simulink model "VIPRStEnCtrl"  (R2018b)
settings: Solver=FixedStepDiscrete  StartTime=0.0  StopTime=10.0  FixedStep=0.01  RelTol=1e-3
undefined symbols (not defined in the file or in its folder): data, PassStFtEn_Clear, PassStFtEn_Set, SecRwRtStBkReclnEn_Clear, SecRwRtStBkReclnEn_Set, SecRwRtStFwdBkwdEn_Clear, SecRwRtStFwdBkwdEn_Set, SecRwRtStLgrstUpwdDnwdEn_Clear, SecRwRtStLgrstUpwdDnwdEn_Set, SecRwRtStLtwdRtwdEn_Clear, SecRwRtStLtwdRtwdEn_Set, ThdRwLtStBkReclnEn_Clear, ThdRwLtStBkReclnEn_Set, ThdRwLtStFwdBkwdEn_Clear, ThdRwLtStFwdBkwdEn_Set, ThdRwRtStBkReclnEn_Clear, ThdRwRtStBkReclnEn_Set, ThdRwRtStFwdBkwdEn_Clear, ThdRwRtStFwdBkwdEn_Set
libraries: simulink x1
settings Model: Creator=sn2xws  LastModifiedBy=sn2xws
settings DataIOCC: SaveFormat=StructureWithTime
settings OptimizationCC: DefaultParameterBehavior=Inlined  EnhancedBackFolding=on  PassReuseOutputArgsAs=Individual arguments  ZeroExternalMemoryAtStartup=off  ZeroInternalMemoryAtStartup=off  OptimizeBlockOrder=speed  DifferentSizesBufferReuse=on  OptimizationCustomize=off
settings DebuggingCC: ParameterTunabilityLossMsg=error
settings ModelReferenceCC: ModelReferenceNumInstancesAllowed=Single
settings SFSimCC: MATLABDynamicMemAlloc=off
settings RTWCC: SystemTargetFile=autosar.tlc  GenCodeOnly=on  TemplateMakefile=ert_default_tmf  Description=AUTOSAR  GenerateReport=on  IncludeHyperlinkInReport=on  LaunchReport=on  GenerateTraceInfo=on  GenerateTraceReport=on  GenerateTraceReportSl=on  GenerateTraceReportSf=on  GenerateTraceReportEml=on  GenerateCodeMetricsReport=on
settings CodeAppCC: ForceParamTrailComments=on  IgnoreCustomStorageClasses=off  OperatorAnnotations=on  SimulinkDataObjDesc=on  SFDataObjDesc=on  InsertBlockDesc=on
settings STFCustomTargetCC: TargetLangStandard=C99 (ISO)  MultiwordLength=256  ParMdlRefBuildCompliant=on  CompOptLevelCompliant=on  IncludeMdlTerminateFcn=off  CombineOutputUpdateFcns=on  SuppressErrorStatus=on  ERTCustomFileBanners=on  SupportNonFinite=off  SupportComplex=off  SupportContinuousTime=off  SupportNonInlinedSFcns=off  RemoveResetFunc=on  MATLABClassNameForMDSCustomization=Simulink.SoftwareTarget.ERTCustomization  AutosarCompliant=on  UseToolchainInfoCompliant=on  LookupTableObjectStructAxisOrder=2,1,3,4,...  LUTObjectStructOrderEvenSpacing=Size,Table,Breakpoints  SystemTargetFile=autosar.tlc
settings ERTTargetCC: TargetLangStandard=C99 (ISO)  ConcurrentExecutionCompliant=off  IncludeMdlTerminateFcn=off  SuppressErrorStatus=on  SupportNonFinite=off  SupportComplex=off  ModelStepFunctionPrototypeControlCompliant=off  CPPClassGenCompliant=off  AutosarCompliant=on  LookupTableObjectStructAxisOrder=2,1,3,4,...  LUTObjectStructOrderEvenSpacing=Size,Table,Breakpoints  InlinedParameterPlacement=NonHierarchical  ERTCustomFileTemplate=example_file_process.tlc  ERTFilePackagingFormat=Compact

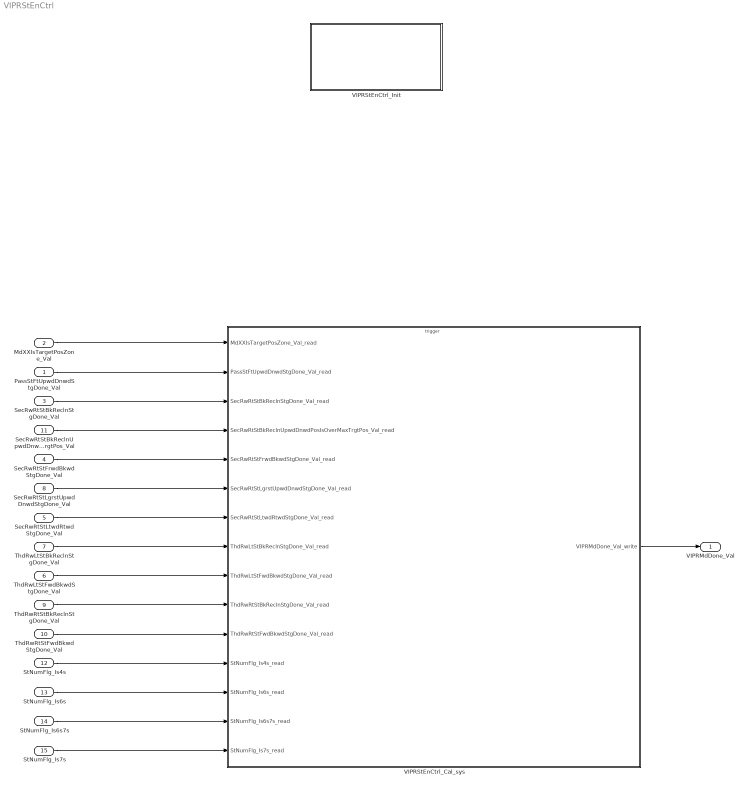
== system VIPRStEnCtrl ==
  PassStFtUpwdDnwdStgDone_Val : Inport  OutDataTypeStr=boolean  PortDimensions=1
  MdXXIsTargetPosZone_Val : Inport  Port=2  OutDataTypeStr=uint32  PortDimensions=1
  SecRwRtStBkReclnStgDone_Val : Inport  Port=3  OutDataTypeStr=boolean  PortDimensions=1
  SecRwRtStFrwdBkwdStgDone_Val : Inport  Port=4  OutDataTypeStr=boolean  PortDimensions=1
  SecRwRtStLtwdRtwdStgDone_Val : Inport  Port=5  OutDataTypeStr=boolean  PortDimensions=1
  ThdRwLtStFwdBkwdStgDone_Val : Inport  Port=6  OutDataTypeStr=boolean  PortDimensions=1
  ThdRwLtStBkReclnStgDone_Val : Inport  Port=7  OutDataTypeStr=boolean  PortDimensions=1
  SecRwRtStLgrstUpwdDnwdStgDone_Val : Inport  Port=8  OutDataTypeStr=boolean  PortDimensions=1
  ThdRwRtStBkReclnStgDone_Val : Inport  Port=9  OutDataTypeStr=boolean  PortDimensions=1
  ThdRwRtStFwdBkwdStgDone_Val : Inport  Port=10  OutDataTypeStr=boolean  PortDimensions=1
  SecRwRtStBkReclnUpwdDnwdPosIsOverMaxTrgtPos_Val : Inport  Port=11  OutDataTypeStr=boolean  PortDimensions=1
  StNumFlg_Is4s : Inport  Port=12  OutDataTypeStr=boolean  PortDimensions=1
  StNumFlg_Is6s : Inport  Port=13  OutDataTypeStr=boolean  PortDimensions=1
  StNumFlg_Is6s7s : Inport  Port=14  OutDataTypeStr=boolean  PortDimensions=1
  StNumFlg_Is7s : Inport  Port=15  OutDataTypeStr=boolean  PortDimensions=1
  VIPRStEnCtrl_Cal_sys : Subsystem
  VIPRStEnCtrl_Init : Subsystem
  VIPRMdDone_Val : Outport  OutDataTypeStr=uint8  PortDimensions=1
  wires:
  VIPRStEnCtrl_Cal_sys/1(VIPRMdDone_Val_write) -> VIPRMdDone_Val/1
  SecRwRtStBkReclnUpwdDnwdPosIsOverMaxTrgtPos_Val/1 -> VIPRStEnCtrl_Cal_sys/4(SecRwRtStBkReclnUpwdDnwdPosIsOverMaxTrgtPos_Val_read)
  MdXXIsTargetPosZone_Val/1 -> VIPRStEnCtrl_Cal_sys/1(MdXXIsTargetPosZone_Val_read)
  ThdRwRtStBkReclnStgDone_Val/1 -> VIPRStEnCtrl_Cal_sys/10(ThdRwRtStBkReclnStgDone_Val_read)
  ThdRwRtStFwdBkwdStgDone_Val/1 -> VIPRStEnCtrl_Cal_sys/11(ThdRwRtStFwdBkwdStgDone_Val_read)
  ThdRwLtStBkReclnStgDone_Val/1 -> VIPRStEnCtrl_Cal_sys/8(ThdRwLtStBkReclnStgDone_Val_read)
  ThdRwLtStFwdBkwdStgDone_Val/1 -> VIPRStEnCtrl_Cal_sys/9(ThdRwLtStFwdBkwdStgDone_Val_read)
  SecRwRtStLtwdRtwdStgDone_Val/1 -> VIPRStEnCtrl_Cal_sys/7(SecRwRtStLtwdRtwdStgDone_Val_read)
  SecRwRtStLgrstUpwdDnwdStgDone_Val/1 -> VIPRStEnCtrl_Cal_sys/6(SecRwRtStLgrstUpwdDnwdStgDone_Val_read)
  SecRwRtStFrwdBkwdStgDone_Val/1 -> VIPRStEnCtrl_Cal_sys/5(SecRwRtStFrwdBkwdStgDone_Val_read)
  SecRwRtStBkReclnStgDone_Val/1 -> VIPRStEnCtrl_Cal_sys/3(SecRwRtStBkReclnStgDone_Val_read)
  PassStFtUpwdDnwdStgDone_Val/1 -> VIPRStEnCtrl_Cal_sys/2(PassStFtUpwdDnwdStgDone_Val_read)
  StNumFlg_Is4s/1 -> VIPRStEnCtrl_Cal_sys/12(StNumFlg_Is4s_read)
  StNumFlg_Is6s/1 -> VIPRStEnCtrl_Cal_sys/13(StNumFlg_Is6s_read)
  StNumFlg_Is6s7s/1 -> VIPRStEnCtrl_Cal_sys/14(StNumFlg_Is6s7s_read)
  StNumFlg_Is7s/1 -> VIPRStEnCtrl_Cal_sys/15(StNumFlg_Is7s_read)

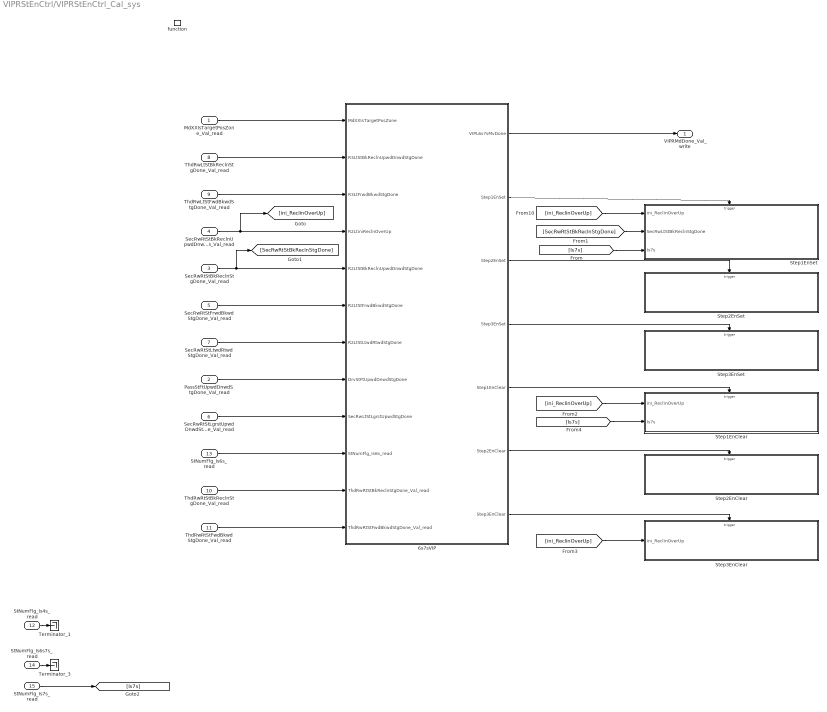
== system VIPRStEnCtrl/VIPRStEnCtrl_Cal_sys ==
  MdXXIsTargetPosZone_Val_read : Inport
  PassStFtUpwdDnwdStgDone_Val_read : Inport  Port=2
  SecRwRtStBkReclnStgDone_Val_read : Inport  Port=3
  SecRwRtStBkReclnUpwdDnwdPosIsOverMaxTrgtPos_Val_read : Inport  Port=4
  SecRwRtStFrwdBkwdStgDone_Val_read : Inport  Port=5
  SecRwRtStLgrstUpwdDnwdStgDone_Val_read : Inport  Port=6
  SecRwRtStLtwdRtwdStgDone_Val_read : Inport  Port=7
  ThdRwLtStBkReclnStgDone_Val_read : Inport  Port=8
  ThdRwLtStFwdBkwdStgDone_Val_read : Inport  Port=9
  ThdRwRtStBkReclnStgDone_Val_read : Inport  Port=10
  ThdRwRtStFwdBkwdStgDone_Val_read : Inport  Port=11
  StNumFlg_Is4s_read : Inport  Port=12
  StNumFlg_Is6s_read : Inport  Port=13
  StNumFlg_Is6s7s_read : Inport  Port=14
  StNumFlg_Is7s_read : Inport  Port=15
  function : TriggerPort  TriggerType=function-call  IsSimulinkFunction=on  FunctionName=VIPRStEnCtrl_Cal  VariantControl=(inherit)
  6s7sVIP : Subsystem
  Step1EnClear : Subsystem  TreatAsAtomicUnit=on
  Step1EnSet : Subsystem  TreatAsAtomicUnit=on
  Step2EnClear : Subsystem  TreatAsAtomicUnit=on
  Step2EnSet : Subsystem  TreatAsAtomicUnit=on
  Step3EnClear : Subsystem  TreatAsAtomicUnit=on
  Step3EnSet : Subsystem  TreatAsAtomicUnit=on
  Terminator_1 : Terminator
  Terminator_3 : Terminator
  VIPRMdDone_Val_write : Outport
      settings: EnsureOutportIsVirtual=on
  wires:
  6s7sVIP/1(VIPL6s7sMvDone) -> VIPRMdDone_Val_write/1
  MdXXIsTargetPosZone_Val_read/1 -> 6s7sVIP/1(MdXXIsTargetPosZone)
  ThdRwLtStBkReclnStgDone_Val_read/1 -> 6s7sVIP/2(R3LtStBkReclnUpwdDnwdStgDone)
  ThdRwLtStFwdBkwdStgDone_Val_read/1 -> 6s7sVIP/3(R3LtFrwdBkwdStgDone)
  SecRwRtStBkReclnUpwdDnwdPosIsOverMaxTrgtPos_Val_read/1 -> [ini_ReclinOverUp], 6s7sVIP/4(R2LtiniReclnOverUp)
  SecRwRtStBkReclnStgDone_Val_read/1 -> [SecRwRtStBkReclnStgDone], 6s7sVIP/5(R2LtStBkReclnUpwdDnwdStgDone)
  SecRwRtStFrwdBkwdStgDone_Val_read/1 -> 6s7sVIP/6(R2LtStFrwdBkwdStgDone)
  SecRwRtStLtwdRtwdStgDone_Val_read/1 -> 6s7sVIP/7(R2LtStLtwdRtwdStgDone)
  PassStFtUpwdDnwdStgDone_Val_read/1 -> 6s7sVIP/8(DrvStFtUpwdDnwdStgDone)
  SecRwRtStLgrstUpwdDnwdStgDone_Val_read/1 -> 6s7sVIP/9(SecRwLtStLgrstUpwdStgDone)
  ThdRwRtStBkReclnStgDone_Val_read/1 -> 6s7sVIP/11(ThdRwRtStBkReclnStgDone_Val_read)
  ThdRwRtStFwdBkwdStgDone_Val_read/1 -> 6s7sVIP/12(ThdRwRtStFwdBkwdStgDone_Val_read)
  6s7sVIP/6(Step2EnClear) -> Step2EnClear/Trigger
  [ini_ReclinOverUp] -> Step1EnSet/1(ini_ReclinOverUp)
  [ini_ReclinOverUp] -> Step3EnClear/1(ini_ReclinOverUp)
  [ini_ReclinOverUp] -> Step1EnClear/1(ini_ReclinOverUp)
  6s7sVIP/3(Step2EnSet) -> Step2EnSet/Trigger
  [Is7s] -> Step1EnClear/2(Is7s)
  [Is7s] -> Step1EnSet/3(Is7s)
  6s7sVIP/5(Step1EnClear) -> Step1EnClear/Trigger
  [SecRwRtStBkReclnStgDone] -> Step1EnSet/2(SecRwLtStBkReclnStgDone)
  6s7sVIP/2(Step1EnSet) -> Step1EnSet/Trigger
  6s7sVIP/4(Step3EnSet) -> Step3EnSet/Trigger
  6s7sVIP/7(Step3EnClear) -> Step3EnClear/Trigger
  StNumFlg_Is4s_read/1 -> Terminator_1/1
  StNumFlg_Is6s7s_read/1 -> Terminator_3/1
  StNumFlg_Is7s_read/1 -> [Is7s]
  StNumFlg_Is6s_read/1 -> 6s7sVIP/10(StNumFlg_Is6s_read)

== system VIPRStEnCtrl/VIPRStEnCtrl_Init ==
  Event Listener : EventListener  EventName=reset

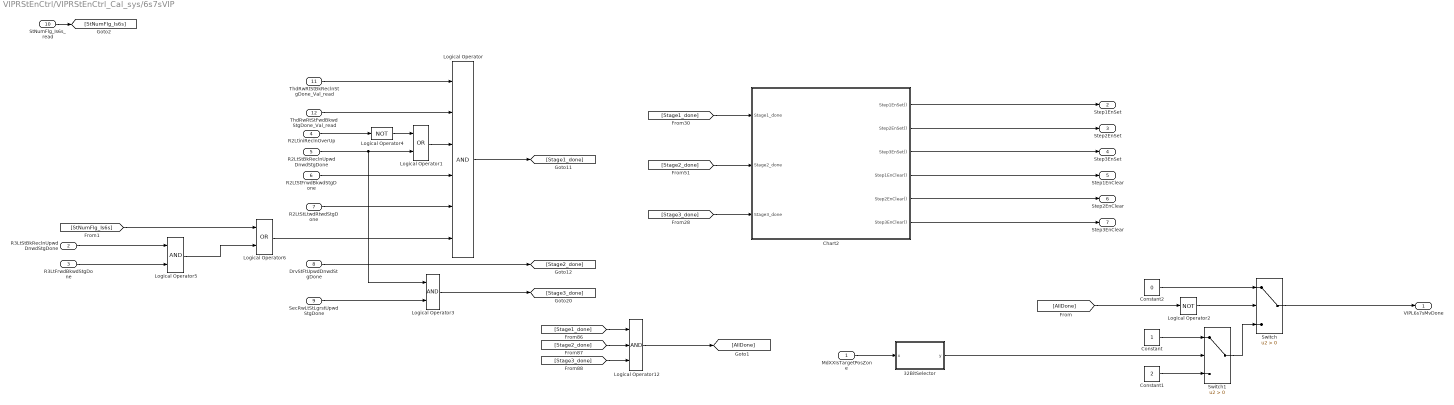
== system VIPRStEnCtrl/VIPRStEnCtrl_Cal_sys/6s7sVIP ==
  MdXXIsTargetPosZone : Inport
  R3LtStBkReclnUpwdDnwdStgDone : Inport  Port=2
  R3LtFrwdBkwdStgDone : Inport  Port=3
  R2LtiniReclnOverUp : Inport  Port=4
  R2LtStBkReclnUpwdDnwdStgDone : Inport  Port=5
  R2LtStFrwdBkwdStgDone : Inport  Port=6
  R2LtStLtwdRtwdStgDone : Inport  Port=7
  DrvStFtUpwdDnwdStgDone : Inport  Port=8
  SecRwLtStLgrstUpwdStgDone : Inport  Port=9
  StNumFlg_Is6s_read : Inport  Port=10
  ThdRwRtStBkReclnStgDone_Val_read : Inport  Port=11
  ThdRwRtStFwdBkwdStgDone_Val_read : Inport  Port=12
  32BitSelector : Subsystem  mask(32 Bit Selector){BitNum=11}
      mask prompts: BitNum "Select Bit Number"
      mask help: Allows selection of a particular bit (0-31) out of a packed word up to 32 bits long. Output will be true if the bit number selected via the mask parameter is equal to one.
      mask TypeOptions BitNum: 0 | 1 | 2 | 3 | 4 | 5 | 6 | 7 | 8 | 9 | 10 | 11 | 12 | 13 | 14 | 15 | 16 | 17 | 18 | 19 | 20 | 21 | 22 | 23 | 24 | 25 | 26 | 27 | 28 | 29 | 30 | 31
      mask Display:
      | text(0.5, 0.8,'BIT','horizontalAlignment','center')
      | text(0.5, 0.5,'SELECTOR','horizontalAlignment','center')
      | text(0.5, 0.2,['-- Bit ',char(get_param(gcb,'BitNum')),' --'],'horizontalAlignment','center')
  Chart2 : Stateflow chart  TreatAsAtomicUnit=on
  Constant : Constant  OutDataTypeStr=uint8
  Constant1 : Constant  Value=2  OutDataTypeStr=uint8
  Constant2 : Constant  Value=0  OutDataTypeStr=uint8
  Logical Operator : Logic  Inputs=6  AllPortsSameDT=off  OutDataTypeStr=boolean
  Logical Operator1 : Logic  Operator=OR  AllPortsSameDT=off  OutDataTypeStr=boolean
  Logical Operator12 : Logic  Inputs=3  AllPortsSameDT=off  OutDataTypeStr=boolean
  Logical Operator2 : Logic  Operator=NOT  AllPortsSameDT=off  OutDataTypeStr=boolean
  Logical Operator3 : Logic  AllPortsSameDT=off  OutDataTypeStr=boolean
  Logical Operator4 : Logic  Operator=NOT  AllPortsSameDT=off  OutDataTypeStr=boolean
  Logical Operator5 : Logic  AllPortsSameDT=off  OutDataTypeStr=boolean
  Logical Operator6 : Logic  Operator=OR  AllPortsSameDT=off  OutDataTypeStr=boolean
  Switch : Switch  Criteria=u2 > Threshold
  Switch1 : Switch  Criteria=u2 > Threshold
  VIPL6s7sMvDone : Outport
  Step1EnSet : Outport  Port=2
  Step2EnSet : Outport  Port=3
  Step3EnSet : Outport  Port=4
  Step1EnClear : Outport  Port=5
  Step2EnClear : Outport  Port=6
  Step3EnClear : Outport  Port=7
  wires:
  [Stage1_done] -> Chart2/1(Stage1_done)
  SecRwLtStLgrstUpwdStgDone/1 -> Logical Operator3/2
  Logical Operator4/1 -> Logical Operator1/1
  [Stage3_done] -> Logical Operator12/3
  [Stage2_done] -> Chart2/2(Stage2_done)
  R2LtStBkReclnUpwdDnwdStgDone/1 -> Logical Operator1/2, Logical Operator3/1
  Logical Operator1/1 -> Logical Operator/3
  Logical Operator/1 -> [Stage1_done]
  Logical Operator3/1 -> [Stage3_done]
  R2LtiniReclnOverUp/1 -> Logical Operator4/1
  R2LtStFrwdBkwdStgDone/1 -> Logical Operator/4
  DrvStFtUpwdDnwdStgDone/1 -> [Stage2_done]
  MdXXIsTargetPosZone/1 -> 32BitSelector/1(x)
  Logical Operator12/1 -> [AllDone]
  [Stage2_done] -> Logical Operator12/2
  R2LtStLtwdRtwdStgDone/1 -> Logical Operator/5
  [Stage1_done] -> Logical Operator12/1
  [Stage3_done] -> Chart2/3(Stage3_done)
  Chart2/1(Step1EnSet()) -> Step1EnSet/1
  Chart2/2(Step2EnSet()) -> Step2EnSet/1
  Chart2/3(Step3EnSet()) -> Step3EnSet/1
  Chart2/4(Step1EnClear()) -> Step1EnClear/1
  Chart2/5(Step2EnClear()) -> Step2EnClear/1
  Chart2/6(Step3EnClear()) -> Step3EnClear/1
  Switch1/1 -> Switch/3
  Switch/1 -> VIPL6s7sMvDone/1
  StNumFlg_Is6s_read/1 -> [StNumFlg_Is6s]
  [StNumFlg_Is6s] -> Logical Operator6/1
  ThdRwRtStBkReclnStgDone_Val_read/1 -> Logical Operator/1
  ThdRwRtStFwdBkwdStgDone_Val_read/1 -> Logical Operator/2
  R3LtFrwdBkwdStgDone/1 -> Logical Operator5/2
  R3LtStBkReclnUpwdDnwdStgDone/1 -> Logical Operator5/1
  Logical Operator5/1 -> Logical Operator6/2
  Logical Operator6/1 -> Logical Operator/6
  Constant2/1 -> Switch/1
  Constant1/1 -> Switch1/3
  Constant/1 -> Switch1/1
  Logical Operator2/1 -> Switch/2
  [AllDone] -> Logical Operator2/1
  32BitSelector/1(y) -> Switch1/2

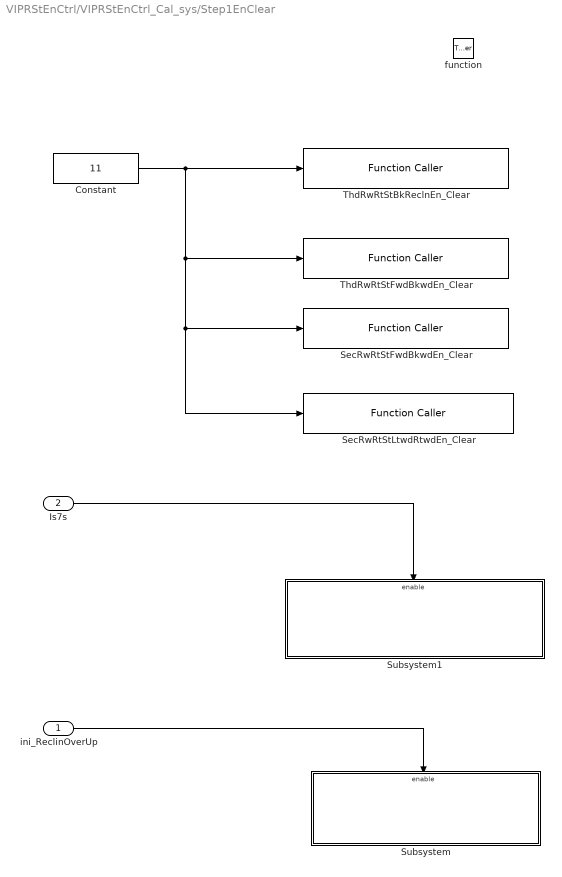
== system VIPRStEnCtrl/VIPRStEnCtrl_Cal_sys/Step1EnClear ==
  ini_ReclinOverUp : Inport
  Is7s : Inport  Port=2
  function : TriggerPort  TriggerType=function-call  VariantControl=Variant
  Constant : Constant  Value=11  OutDataTypeStr=uint8
  SecRwRtStFwdBkwdEn_Clear : FunctionCaller  FunctionPrototype=SecRwRtStFwdBkwdEn_Clear(data)  InputArgumentSpecifications=uint8(1)
  SecRwRtStLtwdRtwdEn_Clear : FunctionCaller  FunctionPrototype=SecRwRtStLtwdRtwdEn_Clear(data)  InputArgumentSpecifications=uint8(1)
  Subsystem : Subsystem
  Subsystem1 : Subsystem
  ThdRwRtStBkReclnEn_Clear : FunctionCaller  FunctionPrototype=ThdRwRtStBkReclnEn_Clear(data)  InputArgumentSpecifications=uint8(1)
  ThdRwRtStFwdBkwdEn_Clear : FunctionCaller  FunctionPrototype=ThdRwRtStFwdBkwdEn_Clear(data)  InputArgumentSpecifications=uint8(1)
  wires:
  Constant/1 -> ThdRwRtStFwdBkwdEn_Clear/1, SecRwRtStLtwdRtwdEn_Clear/1, SecRwRtStFwdBkwdEn_Clear/1, ThdRwRtStBkReclnEn_Clear/1
  ini_ReclinOverUp/1 -> Subsystem/Enable
  Is7s/1 -> Subsystem1/Enable

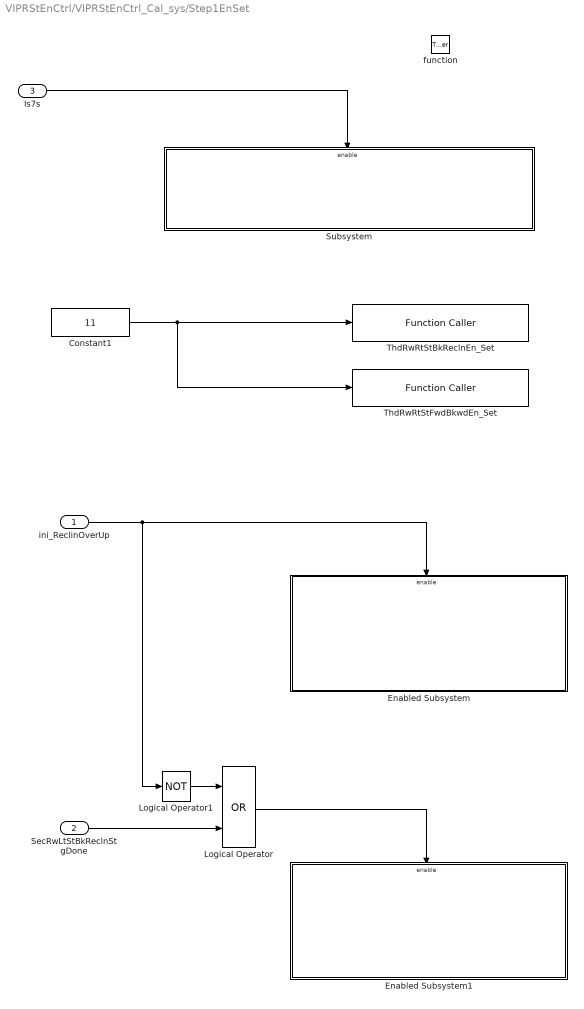
== system VIPRStEnCtrl/VIPRStEnCtrl_Cal_sys/Step1EnSet ==
  ini_ReclinOverUp : Inport
  SecRwLtStBkReclnStgDone : Inport  Port=2
  Is7s : Inport  Port=3
  function : TriggerPort  TriggerType=function-call  VariantControl=Variant
  Constant1 : Constant  Value=11  OutDataTypeStr=uint8
  Enabled Subsystem : Subsystem  TreatAsAtomicUnit=on
  Enabled Subsystem1 : Subsystem  TreatAsAtomicUnit=on
  Logical Operator : Logic  Operator=OR  AllPortsSameDT=off  OutDataTypeStr=boolean
  Logical Operator1 : Logic  Operator=NOT  AllPortsSameDT=off  OutDataTypeStr=boolean
  Subsystem : Subsystem
  ThdRwRtStBkReclnEn_Set : FunctionCaller  FunctionPrototype=ThdRwRtStBkReclnEn_Set(data)  InputArgumentSpecifications=uint8(1)
  ThdRwRtStFwdBkwdEn_Set : FunctionCaller  FunctionPrototype=ThdRwRtStFwdBkwdEn_Set(data)  InputArgumentSpecifications=uint8(1)
  wires:
  ini_ReclinOverUp/1 -> Logical Operator1/1, Enabled Subsystem/Enable
  SecRwLtStBkReclnStgDone/1 -> Logical Operator/2
  Logical Operator1/1 -> Logical Operator/1
  Logical Operator/1 -> Enabled Subsystem1/Enable
  Constant1/1 -> ThdRwRtStFwdBkwdEn_Set/1, ThdRwRtStBkReclnEn_Set/1
  Is7s/1 -> Subsystem/Enable

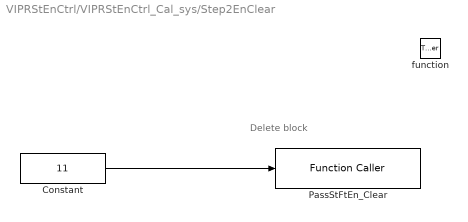
== system VIPRStEnCtrl/VIPRStEnCtrl_Cal_sys/Step2EnClear ==
  note: Delete block
  function : TriggerPort  TriggerType=function-call  VariantControl=Variant
  Constant : Constant  Value=11  OutDataTypeStr=uint8
  PassStFtEn_Clear : FunctionCaller  FunctionPrototype=PassStFtEn_Clear(data)  InputArgumentSpecifications=uint8(1)
  wires:
  Constant/1 -> PassStFtEn_Clear/1

== system VIPRStEnCtrl/VIPRStEnCtrl_Cal_sys/Step2EnSet ==
  function : TriggerPort  TriggerType=function-call  VariantControl=Variant
  Constant : Constant  Value=11  OutDataTypeStr=uint8
  PassStFtEn_Set : FunctionCaller  FunctionPrototype=PassStFtEn_Set(data)  InputArgumentSpecifications=uint8(1)
  wires:
  Constant/1 -> PassStFtEn_Set/1

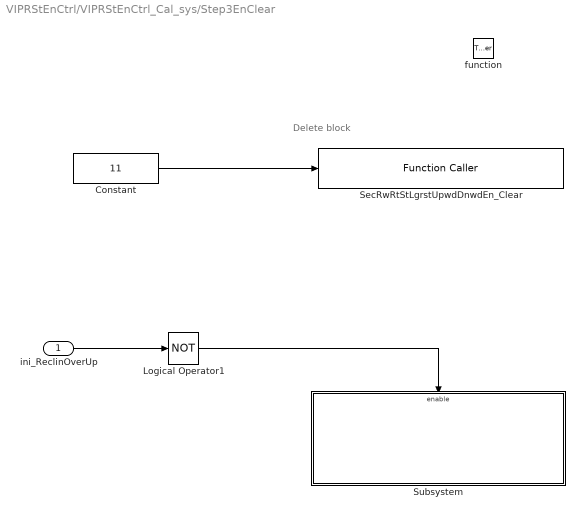
== system VIPRStEnCtrl/VIPRStEnCtrl_Cal_sys/Step3EnClear ==
  note: Delete block
  ini_ReclinOverUp : Inport
  function : TriggerPort  TriggerType=function-call  VariantControl=Variant
  Constant : Constant  Value=11  OutDataTypeStr=uint8
  Logical Operator1 : Logic  Operator=NOT  AllPortsSameDT=off  OutDataTypeStr=boolean
  SecRwRtStLgrstUpwdDnwdEn_Clear : FunctionCaller  FunctionPrototype=SecRwRtStLgrstUpwdDnwdEn_Clear(data)  InputArgumentSpecifications=uint8(1)
  Subsystem : Subsystem
  wires:
  Constant/1 -> SecRwRtStLgrstUpwdDnwdEn_Clear/1
  ini_ReclinOverUp/1 -> Logical Operator1/1
  Logical Operator1/1 -> Subsystem/Enable

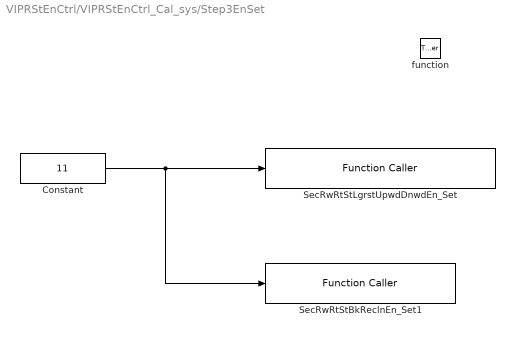
== system VIPRStEnCtrl/VIPRStEnCtrl_Cal_sys/Step3EnSet ==
  function : TriggerPort  TriggerType=function-call  VariantControl=Variant
  Constant : Constant  Value=11  OutDataTypeStr=uint8
  SecRwRtStBkReclnEn_Set1 : FunctionCaller  FunctionPrototype=SecRwRtStBkReclnEn_Set(data)  InputArgumentSpecifications=uint8(1)
  SecRwRtStLgrstUpwdDnwdEn_Set : FunctionCaller  FunctionPrototype=SecRwRtStLgrstUpwdDnwdEn_Set(data)  InputArgumentSpecifications=uint8(1)
  wires:
  Constant/1 -> SecRwRtStLgrstUpwdDnwdEn_Set/1, SecRwRtStBkReclnEn_Set1/1

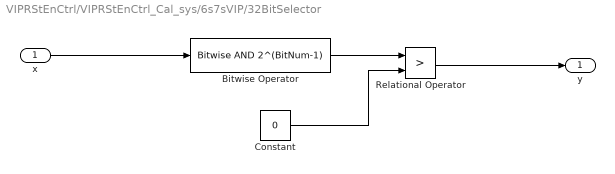
== system VIPRStEnCtrl/VIPRStEnCtrl_Cal_sys/6s7sVIP/32BitSelector ==
  x : Inport
  Bitwise Operator : simulink/Logic and Bit Operations/Bitwise Operator  logicop=AND  UseBitMask=on  BitMask=2^(BitNum-1)  BitMaskRealWorld=Stored Integer
  Constant : Constant  Value=0  OutDataTypeStr=uint32
  Relational Operator : RelationalOperator  Operator=>  OutDataTypeStr=boolean  RndMeth=Simplest
  y : Outport
  wires:
  Relational Operator/1 -> y/1
  Constant/1 -> Relational Operator/2
  x/1 -> Bitwise Operator/1
  Bitwise Operator/1 -> Relational Operator/1

== system VIPRStEnCtrl/VIPRStEnCtrl_Cal_sys/Step1EnClear/Subsystem ==
  Enable : EnablePort
  Constant1 : Constant  Value=11  OutDataTypeStr=uint8
  SecRwRtStBkReclnEn_Clear : FunctionCaller  FunctionPrototype=SecRwRtStBkReclnEn_Clear(data)  InputArgumentSpecifications=uint8(1)
  wires:
  Constant1/1 -> SecRwRtStBkReclnEn_Clear/1

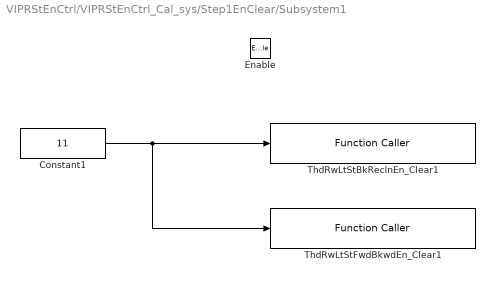
== system VIPRStEnCtrl/VIPRStEnCtrl_Cal_sys/Step1EnClear/Subsystem1 ==
  Enable : EnablePort
  Constant1 : Constant  Value=11  OutDataTypeStr=uint8
  ThdRwLtStBkReclnEn_Clear1 : FunctionCaller  FunctionPrototype=ThdRwLtStBkReclnEn_Clear(data)  InputArgumentSpecifications=uint8(1)
  ThdRwLtStFwdBkwdEn_Clear1 : FunctionCaller  FunctionPrototype=ThdRwLtStFwdBkwdEn_Clear(data)  InputArgumentSpecifications=uint8(1)
  wires:
  Constant1/1 -> ThdRwLtStBkReclnEn_Clear1/1, ThdRwLtStFwdBkwdEn_Clear1/1

== system VIPRStEnCtrl/VIPRStEnCtrl_Cal_sys/Step1EnSet/Enabled Subsystem ==
  Enable : EnablePort
  Constant : Constant  Value=11  OutDataTypeStr=uint8
  SecRwRtStBkReclnEn_Set : FunctionCaller  FunctionPrototype=SecRwRtStBkReclnEn_Set(data)  InputArgumentSpecifications=uint8(1)
  wires:
  Constant/1 -> SecRwRtStBkReclnEn_Set/1

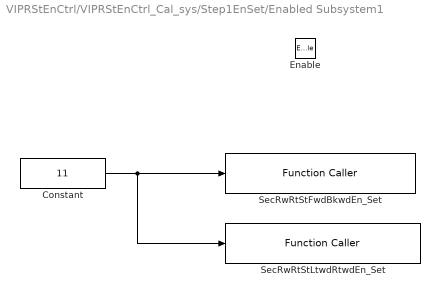
== system VIPRStEnCtrl/VIPRStEnCtrl_Cal_sys/Step1EnSet/Enabled Subsystem1 ==
  Enable : EnablePort
  Constant : Constant  Value=11  OutDataTypeStr=uint8
  SecRwRtStFwdBkwdEn_Set : FunctionCaller  FunctionPrototype=SecRwRtStFwdBkwdEn_Set(data)  InputArgumentSpecifications=uint8(1)
  SecRwRtStLtwdRtwdEn_Set : FunctionCaller  FunctionPrototype=SecRwRtStLtwdRtwdEn_Set(data)  InputArgumentSpecifications=uint8(1)
  wires:
  Constant/1 -> SecRwRtStLtwdRtwdEn_Set/1, SecRwRtStFwdBkwdEn_Set/1

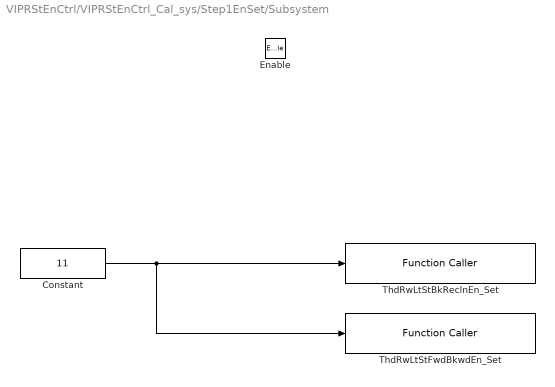
== system VIPRStEnCtrl/VIPRStEnCtrl_Cal_sys/Step1EnSet/Subsystem ==
  Enable : EnablePort
  Constant : Constant  Value=11  OutDataTypeStr=uint8
  ThdRwLtStBkReclnEn_Set : FunctionCaller  FunctionPrototype=ThdRwLtStBkReclnEn_Set(data)  InputArgumentSpecifications=uint8(1)
  ThdRwLtStFwdBkwdEn_Set : FunctionCaller  FunctionPrototype=ThdRwLtStFwdBkwdEn_Set(data)  InputArgumentSpecifications=uint8(1)
  wires:
  Constant/1 -> ThdRwLtStBkReclnEn_Set/1, ThdRwLtStFwdBkwdEn_Set/1

== system VIPRStEnCtrl/VIPRStEnCtrl_Cal_sys/Step3EnClear/Subsystem ==
  note: Delete block
  Enable : EnablePort
  Constant1 : Constant  Value=11  OutDataTypeStr=uint8
  SecRwRtStBkReclnEn_Clear : FunctionCaller  FunctionPrototype=SecRwRtStBkReclnEn_Clear(data)  InputArgumentSpecifications=uint8(1)
  wires:
  Constant1/1 -> SecRwRtStBkReclnEn_Clear/1

== stateflow chart VIPRStEnCtrl/VIPRStEnCtrl_Cal_sys/6s7sVIP/Chart2 ==
  (default) -> (junction 616)
  (junction 616) -> (junction 618) [order 1] : [!Stage1_done]
  (junction 616) -> (junction 622) [order 2]
  (junction 618) -> (junction 620) : {
      | Step1EnSet;
      | Step2EnClear;
      | Step3EnClear;
      | }
  (junction 622) -> (junction 624) [order 1] : [!Stage2_done]
  (junction 622) -> (junction 629) [order 2]
  (junction 624) -> (junction 626) : {
      | Step1EnClear;
      | Step2EnSet;
      | Step3EnClear;
      | }
  (junction 629) -> (junction 631) [order 1] : [!Stage3_done]
  (junction 629) -> (junction 636) [order 2] : {
      | Step1EnClear;
      | Step2EnClear;
      | Step3EnClear;
      | }
  (junction 631) -> (junction 633) : {
      | Step1EnClear;
      | Step2EnClear;
      | Step3EnSet;
      | }
  (junction 633) -> (junction 636)
  (junction 626) -> (junction 633)
  (junction 620) -> (junction 626)
  (junction 636) -> (junction 639)
  data: Stage1_done input boolean; Stage2_done input boolean; Stage3_done input boolean
  events: Step1EnSet output FUNCTION_CALL_EVENT; Step2EnSet output FUNCTION_CALL_EVENT; Step3EnSet output FUNCTION_CALL_EVENT; Step1EnClear output FUNCTION_CALL_EVENT; Step2EnClear output FUNCTION_CALL_EVENT; Step3EnClear output FUNCTION_CALL_EVENT
